simulink model "MBD_WEEK2_QN2"  (R2020b)
settings: Solver=VariableStepAuto  StartTime=0.0  StopTime=10.0  RelTol=1e-3
values from neighbouring files (symbols this model uses):
  b = 3.5076999999999995E-6    [motor_position_control_variable_data.sldd]
  J = 3.2284E-6    [motor_position_control_variable_data.sldd]
  L = 2.75E-6    [motor_position_control_variable_data.sldd]
  R = 4.0    [motor_position_control_variable_data.sldd]
undefined symbols (not defined in the file or in its folder): K
settings Model: Creator=dell  LastModifiedBy=dell

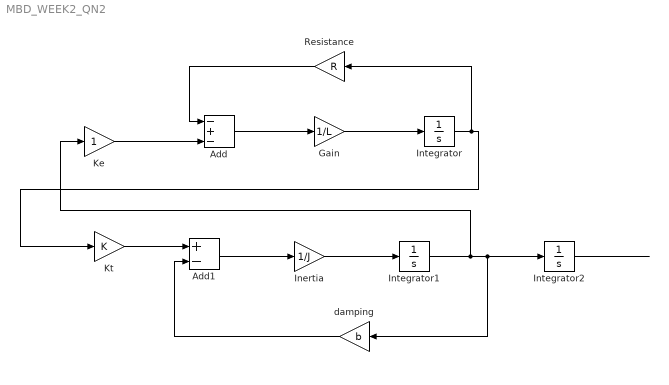
== system MBD_WEEK2_QN2 ==
  Add : Sum  Inputs=-+-
  Add1 : Sum  Inputs=+-
  Gain : Gain  Gain=1/L
  Inertia : Gain  Gain=1/J
  Integrator : Integrator
  Integrator1 : Integrator
  Integrator2 : Integrator
  Ke : Gain
  Kt : Gain  Gain=K
  Resistance : Gain  Gain=R
  damping : Gain  Gain=b
  wires:
  Gain/1 -> Integrator/1
  Integrator/1 -> Resistance/1, Kt/1
  Add1/1 -> Inertia/1
  Integrator1/1 -> Ke/1, damping/1, Integrator2/1
  Integrator2/1 -> ?
  Add/1 -> Gain/1
  Inertia/1 -> Integrator1/1
  Kt/1 -> Add1/1
  damping/1 -> Add1/2
  Resistance/1 -> Add/1
  Ke/1 -> Add/3
  ? -> Add/2
